simulink model "GMCLIB_DecouplingPMSM_BAM_F16"  (Simulink 7.3)
settings: Solver=ode45  StartTime=0.0  StopTime=10.0  RelTol=1e-3
undefined symbols (not defined in the file): f16Kd, f16Kq, s16KdShift, s16KqShift
settings Model: Creator=B17364  LastModifiedBy=B17364

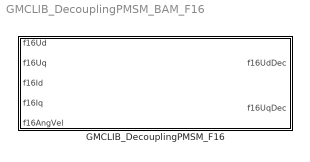
== system GMCLIB_DecouplingPMSM_BAM_F16 ==
  GMCLIB_DecouplingPMSM_F16 : Subsystem  mask(GMCLIB_DecouplingPMSM_F16){f16Kd=f16Kd, s16KdShift=s16KdShift, f16Kq=f16Kq, s16KqShift=s16KqShift}
      mask help: Bit accurate model of decoupling for PMSM model.
      mask init:
      | pos = get_param(gcb, 'Position');width = pos(3) - pos(1); height = pos(4) - pos(2);tX=width/2;tY=height*0.9;
      mask Display: color('black');port_label('input',1,'f16Ud');port_label('input',2,'f16Uq');port_label('input',3,'f16Id');port_label('input',4,'f16Iq');port_label('input',5,'f16AngVel');port_label('output',1,'f16UdDec');port_label('output',2,'f16UqDec');color('black');disp('GMCLIB_DecouplingPMSM_F16');color('blue');text(tX,tY, 'BAM', 'horizontalAlignment', 'center');

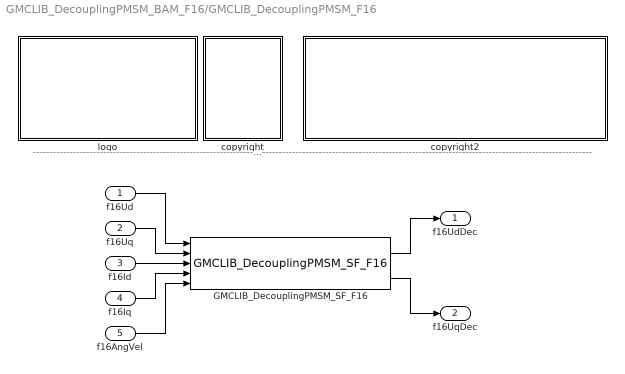
== system GMCLIB_DecouplingPMSM_BAM_F16/GMCLIB_DecouplingPMSM_F16 ==
  note: ---------------------------------------------------------------------------------------------------------------------------------------------------------------------------------------------------
  f16Ud : Inport  OutDataType=fixdt(1, 16)  OutScaling=2^0
  f16Uq : Inport  Port=2  OutDataType=fixdt(1, 16)  OutScaling=2^0
  f16Id : Inport  Port=3  OutDataType=fixdt(1, 16)  OutScaling=2^0
  f16Iq : Inport  Port=4  OutDataType=fixdt(1, 16)  OutScaling=2^0
  f16AngVel : Inport  Port=5  OutDataType=fixdt(1, 16)  OutScaling=2^0
  GMCLIB_DecouplingPMSM_SF_F16 : S-Function  FunctionName=GMCLIB_DecouplingPMSM_SF_F16  Parameters=f16Kd,s16KdShift,f16Kq,s16KqShift  EnableBusSupport=off
  copyright : Subsystem
      mask Display: text(10,90,'FILE:');text(10,75,'DESRIPTION:')text(10,60,'COPYRIGHT:')text(10,45,'VERSION:')text(10,30,'DATE:')
  copyright2 : Subsystem
      mask Display: text(10,90,'GMCLIB_DecouplingPMSM_BAM_F16.mdl');text(10,75,'Decoupling of d and q axis of PMSM model.');text(10,60,'Freescale')text(10,45,'0.1');text(10,30,'14-Sep-2011');
  logo : Subsystem
      mask Display: image(imread('logo.jpg'))
  f16UdDec : Outport  OutDataType=fixdt(1, 16)  OutScaling=2^0
  f16UqDec : Outport  Port=2  OutDataType=fixdt(1, 16)  OutScaling=2^0
  wires:
  f16Ud/1 -> GMCLIB_DecouplingPMSM_SF_F16/1
  f16Uq/1 -> GMCLIB_DecouplingPMSM_SF_F16/2
  f16Id/1 -> GMCLIB_DecouplingPMSM_SF_F16/3
  f16Iq/1 -> GMCLIB_DecouplingPMSM_SF_F16/4
  f16AngVel/1 -> GMCLIB_DecouplingPMSM_SF_F16/5
  GMCLIB_DecouplingPMSM_SF_F16/1 -> f16UdDec/1
  GMCLIB_DecouplingPMSM_SF_F16/2 -> f16UqDec/1

== system GMCLIB_DecouplingPMSM_BAM_F16/GMCLIB_DecouplingPMSM_F16/copyright ==

== system GMCLIB_DecouplingPMSM_BAM_F16/GMCLIB_DecouplingPMSM_F16/copyright2 ==

== system GMCLIB_DecouplingPMSM_BAM_F16/GMCLIB_DecouplingPMSM_F16/logo ==
